simulink model "rgb_arduino1"  (R2019b)
settings: Solver=FixedStepDiscrete  StartTime=0.0  StopTime=inf  FixedStep=0.01  RelTol=1e-3
libraries: arduinolib x6
settings Model: FPTRunName=NoOverride  ExtModeTrigDuration=2  Creator=roslovetspv  LastModifiedBy=bhisma
settings DataIOCC: ReturnWorkspaceOutputs=off
settings OptimizationCC: LifeSpan=1  MaxStackSize=64  EfficientTunableParamExpr=on
settings DebuggingCC: SFUnexpectedBacktrackingDiag=warning  SFNoUnconditionalDefaultTransitionDiag=warning  SFExecutionAtInitializationDiag=none  ArithmeticOperatorsInVariantConditions=warning
settings HardwareCC: ProdBitPerInt=16  ProdBitPerPointer=16  ProdBitPerSizeT=16  ProdBitPerPtrDiffT=16  ProdLargestAtomicFloat=None  ProdWordSize=8  ProdHWDeviceType=Atmel->AVR
settings SFSimCC: SimUseLocalCustomCode=off  MATLABDynamicMemAlloc=off  CustomCodeUndefinedFunction=UseInterfaceOnly
settings RTWCC: SystemTargetFile=ert.tlc  HardwareBoard=Arduino Uno  TLCOptions=-aInlineSetEventsForThisBaseRateFcn=TLC_FALSE -aSuppressMultiTaskScheduler=TLC_FALSE -aRateBasedStepFcn=1  TemplateMakefile=ert_default_tmf  GenerateReport=on  RTWUseLocalCustomCode=off  Toolchain=Arduino AVR  BuildConfiguration=Faster Runs  IncludeHyperlinkInReport=on  LaunchReport=on  GenerateTraceInfo=on  GenerateTraceReport=on  GenerateTraceReportSl=on  GenerateTraceReportSf=on  GenerateTraceReportEml=on
settings CodeAppCC: ForceParamTrailComments=on  IgnoreCustomStorageClasses=off  OperatorAnnotations=on  SimulinkDataObjDesc=on  SFDataObjDesc=on  MATLABFcnDesc=on  InsertBlockDesc=on  StateflowObjectComments=on  MATLABSourceComments=on
settings ERTTargetCC: MultiwordLength=2048  SupportContinuousTime=on  SupportVariableSizeSignals=on
settings ConfigComp: CovMetricSettings=dw  CovHtmlReporting=on  CovSaveCumulativeToWorkspaceVar=on  CovSaveSingleToWorkspaceVar=on  CovExternalEMLEnable=off
settings SimscapeCC: SimscapeNormalizeSystem=off

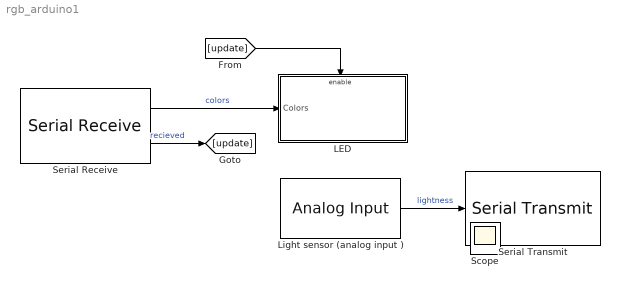
== system rgb_arduino1 ==
  LED : Subsystem  TreatAsAtomicUnit=on
  Light sensor (analog input ) : arduinolib/Analog Input  pinNumber=0  sampleTime=0.07  blockPlatform=arduino
      settings: AttributesFormatString=Ts = %<SampleTime>
  Serial Receive : arduinolib/Serial Receive  isARMArch=off  portNumber=0  DataType=uint8  Datalength=3  SampleTime=0.01  showOutStatus=on  blockPlatform=arduino
      settings: AttributesFormatString=Ts = %<SampleTime>  SourceProductName=Simulink Support Package for Arduino Hardware  SourceProductBaseCode=ARDUINO
  Serial Transmit : arduinolib/Serial Transmit  portNumber=0  sendmode=write  sendformat=Decimal  floatprecision=2  blockPlatform=arduino
      settings: SourceProductName=Simulink Support Package for Arduino Hardware
  Scope : Scope
  wires:
  Serial Receive/1 -> LED/1(Colors)  "colors"
  Light sensor (analog input )/1 -> Serial Transmit/1  "lightness"
  Serial Receive/2 -> [update]  "recieved"
  [update] -> LED/Enable

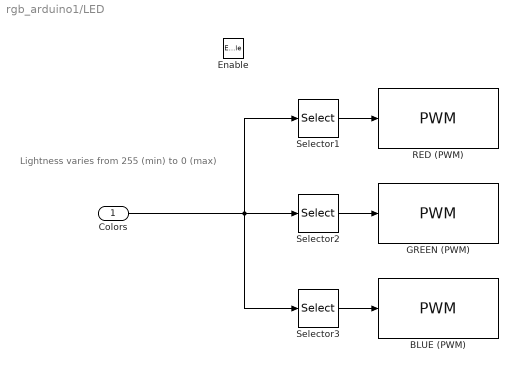
== system rgb_arduino1/LED ==
  note: Lightness varies from 255 (min) to 0 (max)
  Colors : Inport  OutDataTypeStr=uint8
  Enable : EnablePort
  BLUE (PWM) : arduinolib/PWM  pinNumber=11  blockPlatform=arduino
  GREEN (PWM) : arduinolib/PWM  pinNumber=10  blockPlatform=arduino
  RED (PWM) : arduinolib/PWM  pinNumber=9  blockPlatform=arduino
  Selector1 : Selector  InputPortWidth=3  IndexOptions=Index vector (dialog)  Indices=1  OutputSizes=1
  Selector2 : Selector  InputPortWidth=3  IndexOptions=Index vector (dialog)  Indices=2  OutputSizes=1
  Selector3 : Selector  InputPortWidth=3  IndexOptions=Index vector (dialog)  Indices=3  OutputSizes=1
  wires:
  Selector2/1 -> GREEN (PWM)/1
  Selector3/1 -> BLUE (PWM)/1
  Selector1/1 -> RED (PWM)/1
  Colors/1 -> Selector1/1, Selector3/1, Selector2/1
